simulink model "is95fwdchendtoend"  (Simulink 4.00)
settings: Solver=VariableStepDiscrete  SolverMode=SingleTasking  StartTime=0.0  StopTime=600  RelTol=1e-3  AbsTol=1e-6
undefined symbols (not defined in the file): Fs, magnitude
libraries: cdmalib x14, dspsrcs2 x13, dspbuff2 x5, dspxfrm2 x3, dspstat2 x3, dspsnks2 x3, dspmtrx2 x2, commsink x2, commchan x2
settings Model: RequirementInfo=9  Creator=pc  LastModifiedBy=akansal  SaveTime=off  SaveOutput=off  LimitDataPoints=off  ExtModeTrigMode=oneshot  ExtModeArmWhenConnect=off  BlockReductionOpt=off

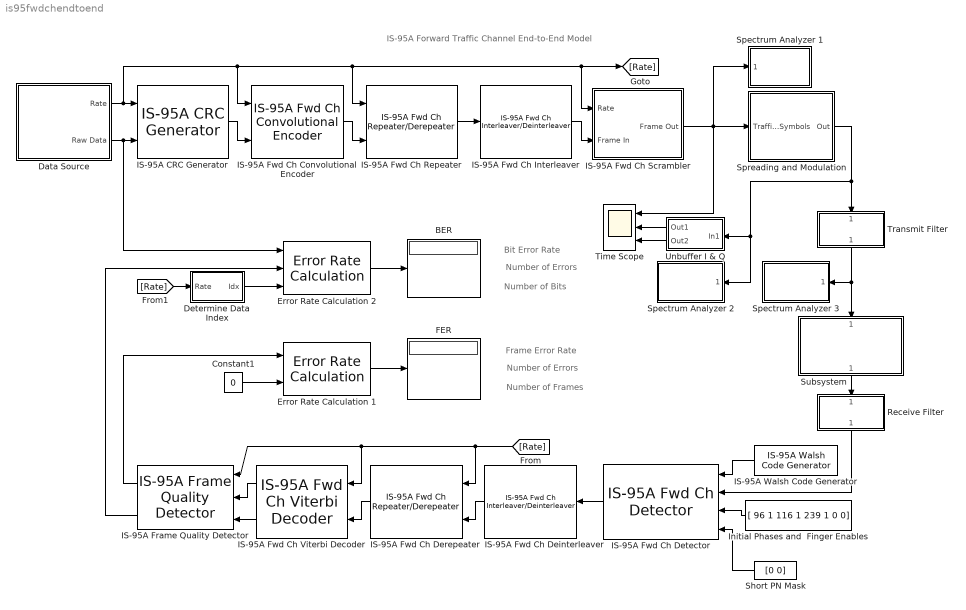
== system is95fwdchendtoend ==
  note: IS-95A Forward Traffic Channel
      | End-to-End Model
  note: Frame Error Rate
  note: Number of Errors
  note: Number of Frames
  note: Bit Error Rate
  note: Number of Errors
  note: Number of Bits
  BER : Display
      settings: Format=short
  Constant1 : Constant  Value=0
  Data Source : Subsystem
      settings: RTWFcnNameOpts=Auto  RTWFileNameOpts=Auto
  Determine Data Index : Subsystem  mask(Determine Data Index){rateSet=Rate Set I}
      mask prompts: rateSet "Rate set:"
      mask help: Deterime index of valid data in the frame based upon rate set and rate input.
      mask init:
      | if(rateSet==1)
      | % --- Rate Set 1
      |    R1F = buffer(1:172,268);
      |    R1H = buffer(1:80,268);
      |    R1Q = buffer(1:40,268);
      |    R1E = buffer(1:16,268);
      |    idxMat = [R1F R1H R1Q R1E];
      | else
      |    % --- Rate Set 2
      |    R2F = [1:268]';
      |    R2H = buffer(1:126,268);
      |    R2Q = buffer(1:56,268);
      |    R2E = buffer(1:22,268);
      |    idxMat = [R2F R2H R2Q R2E];
      | end;
      settings: RTWFcnNameOpts=Auto  RTWFileNameOpts=Auto
      mask StyleString: popup(Rate Set I|Rate Set II)
  Error Rate Calculation 1 : commsink/Error Rate Calculation  N=0  st_delay=4  cp_mode=Entire frame  subframe=[]  PMode=Port  WsName=ErrorVec  RsMode2=off
  Error Rate Calculation 2 : commsink/Error Rate Calculation  N=2*268  st_delay=2*268  cp_mode=Select samples from port  subframe=[]  PMode=Port  WsName=ErrorVec  RsMode2=off
  FER : Display
      settings: Format=short
  IS-95A CRC Generator : cdmalib/IS-95A Common/IS-95A CRC Generator  rate_set=Rate Set I  ch_type=Traffic
  IS-95A Frame Quality Detector : cdmalib/IS-95A Common/IS-95A Frame Quality  Detector  Orientation=left  rateSet=Rate Set I  chType=Traffic  rate2_metric=0.9*1.5  rate3_metric=0.85*1.5
  IS-95A Fwd Ch Convolutional Encoder : cdmalib/IS-95A Base Station Transmitter/IS-95A Fwd Ch Convolutional Encoder  rate_set=Rate Set I  ch_type=Traffic  enc_state=[]
  IS-95A Fwd Ch Deinterleaver : cdmalib/IS-95A Base Station Transmitter/IS-95A Fwd Ch Interleaver//Deinterleaver  Orientation=left  ch_type=Traffic  int_select=Deinterleaver
  IS-95A Fwd Ch Derepeater : cdmalib/IS-95A Base Station Transmitter/IS-95A Fwd Ch Repeater//Derepeater  Orientation=left  rate_set=Rate Set I  ch_type=Traffic  rep_select=Derepeater
  IS-95A Fwd Ch Interleaver : cdmalib/IS-95A Base Station Transmitter/IS-95A Fwd Ch Interleaver//Deinterleaver  ch_type=Traffic  int_select=Interleaver
  IS-95A Fwd Ch Repeater : cdmalib/IS-95A Base Station Transmitter/IS-95A Fwd Ch Repeater//Derepeater  rate_set=Rate Set I  ch_type=Traffic  rep_select=Repeater
  IS-95A Fwd Ch Scrambler : Subsystem  mask(IS-95A Fwd Ch Scrambler){rate_set=Rate Set I, chType=Traffic}
      mask prompts: rate_set "Rate Set"; chType "Channel Type"
      mask help: Performs scrambling of the Forward Traffic channel data by the long code and the insertion of power bits in the data.
      settings: RTWFcnNameOpts=Auto  RTWFileNameOpts=Auto
      mask Help: web(cdmaweb);
      mask StyleString: popup(Rate Set I|Rate Set II),popup(Sync|Paging|Traffic)
  IS-95A Fwd Ch Viterbi Decoder : cdmalib/IS-95A Mobile Station Receiver/IS-95A Fwd Ch Viterbi Decoder  Orientation=left  rateSet=Rate Set I  chType=Traffic  traceBackLenRatio=1  decodeLenRatio=1
  IS-95A Fwd Ch Detector : cdmalib/IS-95A Mobile Station Receiver/IS-95A Fwd Ch Detector  Orientation=left  rateSet=Rate Set I  numSymb=1  wlshOrd=6  rake_buff_size=3  rake_oversamp=8  sampTime=1/(50*384)
  IS-95A Walsh Code Generator : cdmalib/IS-95A Common/IS-95A Walsh Code Generator  Orientation=left  wlshOrd=6  wlshIndices=38  st=1/50/384
  Initial Phases and  Finger Enables : Constant  Orientation=left  Value=[ 96 1 116 1 239 1 0 0]
  Receive Filter : Subsystem  Orientation=down  mask{N=1}
      mask prompts: N "Interpolation factor:"
      mask init:
      | load txfiltx8.mat;
      | h = (TxFiltCoefx8*N)/8;
      settings: RTWFcnNameOpts=Auto  RTWFileNameOpts=Auto
      mask Display: plot( 1:prod( size( h)), h);
  Short PN Mask : Constant  Orientation=left  Value=[0 0]
  Spectrum Analyzer 1 : Subsystem
      settings: RTWFcnNameOpts=Auto  RTWFileNameOpts=Auto
      mask Display: disp('Spectrum\nAnalyzer');
  Spectrum Analyzer 2 : Subsystem  Orientation=left
      settings: RTWFcnNameOpts=Auto  RTWFileNameOpts=Auto
      mask Display: disp('Spectrum\nAnalyzer');
  Spectrum Analyzer 3 : Subsystem  Orientation=left
      settings: RTWFcnNameOpts=Auto  RTWFileNameOpts=Auto
      mask Display: disp('Spectrum\nAnalyzer');
  Spreading and Modulation : Subsystem
      settings: RTWFcnNameOpts=Auto  RTWFileNameOpts=Auto
      mask Display: disp('Combine with\nSync & Paging\n---\nSS Modulate')
  Subsystem : Subsystem  Orientation=down
      settings: RTWFcnNameOpts=Auto  RTWFileNameOpts=Auto
      mask Display: disp('Rayleigh Multipath\n and  AWGN\nChannel')
  Time Scope : Scope  NumInputPorts=3
      settings: TimeRange=0.001041666666666667  YMin=-3~-3~-3  YMax=3~3~3  SaveToWorkspace=off  SaveName=ScopeData  DataFormat=Structure  LimitDataPoints=on  MaxDataPoints=5000
  Transmit Filter : Subsystem  Orientation=down  mask{N=8}
      mask prompts: N "Interpolation factor:"
      mask init:
      | load txfiltx8.mat;
      | h = (TxFiltCoefx8*N)/8;
      settings: RTWFcnNameOpts=Auto  RTWFileNameOpts=Auto
      mask Display: plot( 1:prod( size( h)), h);
  Unbuffer I & Q : Subsystem  Orientation=left
      settings: RTWFcnNameOpts=Auto  RTWFileNameOpts=Auto
      mask Display: disp('Unbuffer\nI & Q');
  wires:
  Error Rate Calculation 2/1 -> BER/1
  [Rate] -> Determine Data Index/1(Rate)
  Error Rate Calculation 1/1 -> FER/1
  Constant1/1 -> Error Rate Calculation 1/2
  Determine Data Index/1(Idx) -> Error Rate Calculation 2/3
  Subsystem/1("  ") -> Receive Filter/1("   ")
  Initial Phases and  Finger Enables/1 -> IS-95A Fwd Ch Detector/3
  IS-95A Walsh Code Generator/1 -> IS-95A Fwd Ch Detector/1
  Short PN Mask/1 -> IS-95A Fwd Ch Detector/4
  IS-95A Fwd Ch Deinterleaver/1 -> IS-95A Fwd Ch Derepeater/2
  IS-95A Fwd Ch Derepeater/1 -> IS-95A Fwd Ch Viterbi Decoder/2
  IS-95A Fwd Ch Viterbi Decoder/1 -> IS-95A Frame Quality Detector/2
  IS-95A Fwd Ch Viterbi Decoder/2 -> IS-95A Frame Quality Detector/3
  IS-95A Fwd Ch Detector/1 -> IS-95A Fwd Ch Deinterleaver/1
  Receive Filter/1(" ") -> IS-95A Fwd Ch Detector/2
  IS-95A Frame Quality Detector/1 -> Error Rate Calculation 1/1
  IS-95A Frame Quality Detector/2 -> Error Rate Calculation 2/2
  [Rate] -> IS-95A Fwd Ch Derepeater/1, IS-95A Frame Quality Detector/1, IS-95A Fwd Ch Viterbi Decoder/1
  IS-95A Fwd Ch Repeater/1 -> IS-95A Fwd Ch Interleaver/1
  IS-95A Fwd Ch Convolutional Encoder/1 -> IS-95A Fwd Ch Repeater/2
  Data Source/1(Rate) -> IS-95A Fwd Ch Convolutional Encoder/1, IS-95A Fwd Ch Repeater/1, [Rate], IS-95A Fwd Ch Scrambler/1(Rate), IS-95A CRC Generator/1
  IS-95A Fwd Ch Interleaver/1 -> IS-95A Fwd Ch Scrambler/2(Frame In)
  IS-95A CRC Generator/1 -> IS-95A Fwd Ch Convolutional Encoder/2
  Data Source/2(Raw Data) -> IS-95A CRC Generator/2, Error Rate Calculation 2/1
  IS-95A Fwd Ch Scrambler/1(" Frame Out") -> Spreading and Modulation/1(Traffic Symbols), Spectrum Analyzer 1/1(" "), Time Scope/1
  Spreading and Modulation/1("Out ") -> Transmit Filter/1("   "), Spectrum Analyzer 2/1(" "), Unbuffer I & Q/1(In1)
  Transmit Filter/1(" ") -> Subsystem/1(" "), Spectrum Analyzer 3/1(" ")
  Unbuffer I & Q/1(Out1) -> Time Scope/2
  Unbuffer I & Q/2(Out2) -> Time Scope/3

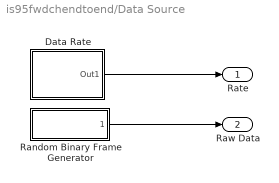
== system is95fwdchendtoend/Data Source ==
  Data Rate : Subsystem  mask{rate=Full}
      mask prompts: rate "Data Rate"
      settings: RTWFcnNameOpts=Auto  RTWFileNameOpts=Auto
      mask StyleString: popup(Full|Half|Quarter|One-Eighth)
      mask Display: disp('Base Station \nTransmitter\nData Rate')
  Random Binary Frame Generator : Subsystem  mask(Random binary frame generator){seed=1234, Ts=1/(50*268), N=268}
      mask prompts: seed "Initial seed:"; Ts "Sample time (sec):"; N "Output frame size:"
      mask help:
      | Generate a random frame of binary integers. The output frame period is
      | (Sample time) * (Output frame size).
      settings: RTWFcnNameOpts=Auto  RTWFileNameOpts=Auto
      mask Display: plot(0,0,100,100,[95,90,90,80,80,60,60,30,30,20,20,10,10,5],[25,25,75,75,25,25,75,75,25,25,75,75,25,25]);
  Rate : Outport  Port=1  InitialOutput=0
  Raw Data : Outport  Port=2  InitialOutput=0
  wires:
  Data Rate/1(Out1) -> Rate/1
  Random Binary Frame Generator/1(" ") -> Raw Data/1

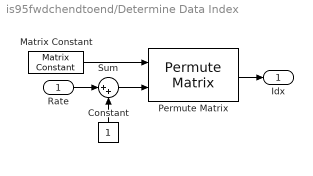
== system is95fwdchendtoend/Determine Data Index ==
  Rate : Inport  Port=1
  Constant : Constant  Orientation=up  Value=1
  Matrix Constant : dspmtrx2/Matrix Constant  M=idxMat
  Permute Matrix : dspmtrx2/Permute Matrix  mode=Columns  errmode=Clip Index  cols=4
  Sum : Sum  Inputs=|++  SaturateOnIntegerOverflow=on
  Idx : Outport  Port=1
  wires:
  Constant/1 -> Sum/2
  Matrix Constant/1 -> Permute Matrix/1
  Permute Matrix/1 -> Idx/1
  Sum/1 -> Permute Matrix/2
  Rate/1 -> Sum/1

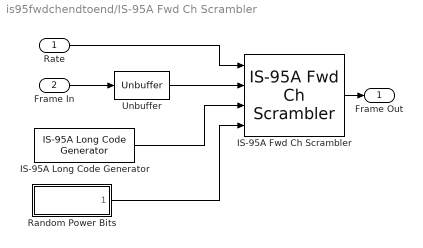
== system is95fwdchendtoend/IS-95A Fwd Ch Scrambler ==
  Rate : Inport  Port=1
  Frame In : Inport  Port=2
  IS-95A Fwd Ch Scrambler : cdmalib/IS-95A Base Station Transmitter/IS-95A Fwd Ch Scrambler  rate_set=Rate Set I  chType=Traffic
  IS-95A Long Code Generator : cdmalib/IS-95A Common/IS-95A Long Code Generator  num_symb=1  tx_lc_dec_ratio=64  tx_lc_init_mask=2^41  tx_lc_init_state=2^41  tx_sample_time=1/(50*384)
  Random Power Bits : Subsystem  mask(Random binary frame generator){seed=956742, Ts=1/50/16, N=1}
      mask prompts: seed "Initial seed:"; Ts "Sample time (sec):"; N "Ouput frame size:"
      settings: RTWFcnNameOpts=Auto  RTWFileNameOpts=Auto
      mask Display: plot(0,0,100,100,[95,90,90,80,80,60,60,30,30,20,20,10,10,5],[25,25,75,75,25,25,75,75,25,25,75,75,25,25]);
  Unbuffer : dspbuff2/Unbuffer  ic=0  num_chans=1
  " Frame Out" : Outport  Port=1  InitialOutput=0
  wires:
  Rate/1 -> IS-95A Fwd Ch Scrambler/1
  IS-95A Fwd Ch Scrambler/1 -> " Frame Out"/1
  Random Power Bits/1(" ") -> IS-95A Fwd Ch Scrambler/4
  Frame In/1 -> Unbuffer/1
  Unbuffer/1 -> IS-95A Fwd Ch Scrambler/2
  IS-95A Long Code Generator/1 -> IS-95A Fwd Ch Scrambler/3

== system is95fwdchendtoend/Receive Filter ==
  "   " : Inport  Port=1
  FIR Interpolation : Subsystem  mask(FIR Interpolation){h=h, L=N, frame=on, numChans=1, framing=Maintain input frame rate}
      mask prompts: h "FIR filter coefficients:"; L "Interpolation factor:"; frame "Frame-based inputs"; numChans "Number of channels:"
      mask help: Upsample input signal by an integer factor, then apply an FIR filter. Implemented using an efficient polyphase interpolation structure. The filter coefficients are scaled by the interpolation factor.
      mask init:
      | outputBufInitCond = 0;
      | [str,numChans] = dspblkupfir('setup1',numChans);
      | [h,framing,str]= dspblkupfir('setup2',h,L,framing);
      settings: RTWFcnNameOpts=Auto  RTWFileNameOpts=Auto
      mask Help: web(dspbhelp);
      mask StyleString: edit,edit,checkbox,edit,popup(Maintain input frame size|Maintain input frame rate)
      mask CallbackString: ||dspblkupfir||
      mask Display: disp(str)
  " " : Outport  Port=1
  wires:
  "   "/1 -> FIR Interpolation/1(in_1)
  FIR Interpolation/1(out_1) -> " "/1

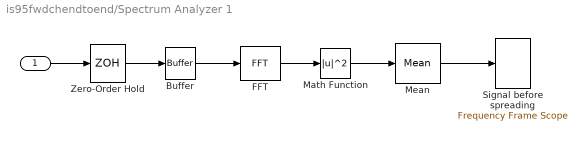
== system is95fwdchendtoend/Spectrum Analyzer 1 ==
  " " : Inport  Port=1
  Buffer : dspbuff2/Buffer  N=1024  V=0  ic=0
  FFT : dspxfrm2/FFT  nchans=1
  Math Function : Math  Operator=magnitude^2  OutputSignalType=auto
  Mean : dspstat2/Mean  run=on  reset=off  frame=off  nchans=1
  Signal before spreading : dspsnks2/Frequency Frame Scope  Domain=Frequency  XLabel=Samples  XUnits=Hertz  XRange=[-Fs/2...Fs/2]  XIncr=-1  YLabel=Magnitude, dB  YUnits=dB  HorizSpan=1  NChans=1  AxisParams=on  FigPos=[339 599 602 134]  AxisGrid=on  AxisZoom=on  FrameNumber=off  AxisLegend=off  Memory=off  LineParams=off
      settings: YMin=-10  YMax=100
  Zero-Order Hold : ZeroOrderHold  SampleTime=1/50/384/64
  wires:
  Zero-Order Hold/1 -> Buffer/1
  " "/1 -> Zero-Order Hold/1
  Buffer/1 -> FFT/1
  FFT/1 -> Math Function/1
  Math Function/1 -> Mean/1
  Mean/1 -> Signal before spreading/1

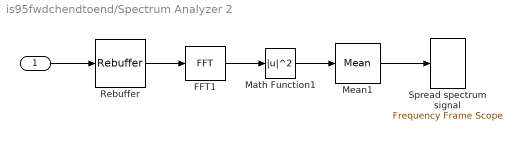
== system is95fwdchendtoend/Spectrum Analyzer 2 ==
  " " : Inport  Port=1
  FFT1 : dspxfrm2/FFT  nchans=1
  Math Function1 : Math  Operator=magnitude^2  OutputSignalType=auto
  Mean1 : dspstat2/Mean  run=on  reset=off  frame=off  nchans=1
  Rebuffer : dspbuff2/Rebuffer  Specify_Out_Size=on  N=1024  V=0  ic=0  frame=on  num_chans=1
  Spread spectrum signal : dspsnks2/Frequency Frame Scope  Domain=Frequency  XLabel=Samples  XUnits=Hertz  XRange=[-Fs/2...Fs/2]  XIncr=-1  YLabel=Magnitude, dB  YUnits=dB  HorizSpan=1  NChans=1  AxisParams=on  FigPos=[339 439 602 134]  AxisGrid=on  AxisZoom=on  FrameNumber=off  AxisLegend=off  Memory=off  LineParams=off
      settings: YMin=-10  YMax=100
  wires:
  " "/1 -> Rebuffer/1
  Rebuffer/1 -> FFT1/1
  Mean1/1 -> Spread spectrum signal/1
  FFT1/1 -> Math Function1/1
  Math Function1/1 -> Mean1/1

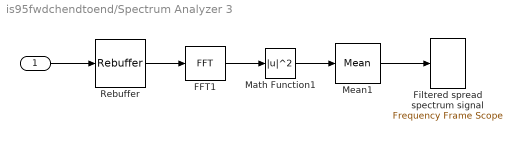
== system is95fwdchendtoend/Spectrum Analyzer 3 ==
  " " : Inport  Port=1
  FFT1 : dspxfrm2/FFT  nchans=1
  Filtered spread spectrum signal : dspsnks2/Frequency Frame Scope  Domain=Frequency  XLabel=Samples  XUnits=Hertz  XRange=[-Fs/2...Fs/2]  XIncr=-1  YLabel=Magnitude, dB  YUnits=dB  HorizSpan=1  NChans=1  AxisParams=on  FigPos=[339 281 602 134]  AxisGrid=on  AxisZoom=on  FrameNumber=off  AxisLegend=off  Memory=off  LineParams=off
      settings: YMin=-10  YMax=100
  Math Function1 : Math  Operator=magnitude^2  OutputSignalType=auto
  Mean1 : dspstat2/Mean  run=on  reset=off  frame=off  nchans=1
  Rebuffer : dspbuff2/Rebuffer  Specify_Out_Size=on  N=8192  V=0  ic=0  frame=on  num_chans=1
  wires:
  Math Function1/1 -> Mean1/1
  FFT1/1 -> Math Function1/1
  Mean1/1 -> Filtered spread spectrum signal/1
  Rebuffer/1 -> FFT1/1
  " "/1 -> Rebuffer/1

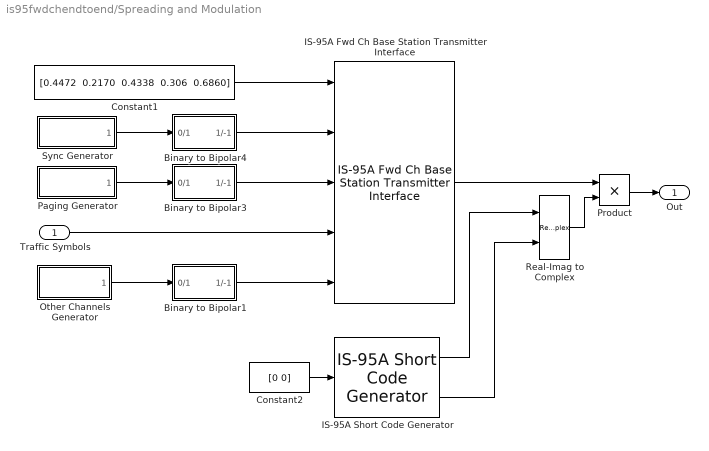
== system is95fwdchendtoend/Spreading and Modulation ==
  Traffic Symbols : Inport  Port=1
  Binary to Bipolar1 : Subsystem
      settings: RTWFcnNameOpts=Auto  RTWFileNameOpts=Auto
      mask Type: Binary to Bipolar Transformation
      mask Description: Binary to Bipolar Transformation.
  Binary to Bipolar3 : Subsystem
      settings: RTWFcnNameOpts=Auto  RTWFileNameOpts=Auto
      mask Type: Binary to Bipolar Transformation
      mask Description: Binary to Bipolar Transformation.
  Binary to Bipolar4 : Subsystem
      settings: RTWFcnNameOpts=Auto  RTWFileNameOpts=Auto
      mask Type: Binary to Bipolar Transformation
      mask Description: Binary to Bipolar Transformation.
  Constant1 : Constant  Value="[0.4472  0.2170  0.4338  0.306  0.6860]"
  Constant2 : Constant  Value=[0 0]
  IS-95A Fwd Ch Base Station Transmitter Interface : cdmalib/IS-95A Base Station Transmitter/IS-95A Fwd Ch Base Station Transmitter Interface  paging_rate=Full  wlshOrd=6  wlsh_indices=[0 32 47 38 23]  sampTime=1/(50*384)
  IS-95A Short Code Generator : cdmalib/IS-95A Common/IS-95A Short Code Generator  numOut=64  sampTime=1/(50*384)
  Other Channels Generator : Subsystem  mask(Random binary frame generator){seed=98767657, Ts=1/(50*384), N=1}
      mask prompts: seed "Initial seed:"; Ts "Sample time (sec):"; N "Output frame size:"
      mask help:
      | Generate a random frame of binary integers. The output frame period is
      | (Sample time) * (Output frame size).
      settings: RTWFcnNameOpts=Auto  RTWFileNameOpts=Auto
      mask Display: plot(0,0,100,100,[95,90,90,80,80,60,60,30,30,20,20,10,10,5],[25,25,75,75,25,25,75,75,25,25,75,75,25,25]);
  Paging Generator : Subsystem  mask(Random binary frame generator){seed=76767, Ts=1/(50*384), N=1}
      mask prompts: seed "Initial seed:"; Ts "Sample time (sec):"; N "Output frame size:"
      mask help:
      | Generate a random frame of binary integers. The output frame period is
      | (Sample time) * (Output frame size).
      settings: RTWFcnNameOpts=Auto  RTWFileNameOpts=Auto
      mask Display: plot(0,0,100,100,[95,90,90,80,80,60,60,30,30,20,20,10,10,5],[25,25,75,75,25,25,75,75,25,25,75,75,25,25]);
  Product : Product  Inputs=2  Multiplication=Element-wise(.*)  SaturateOnIntegerOverflow=on
  Real-Imag to Complex : RealImagToComplex  Input=RealAndImag  ConstantPart=0
  Sync Generator : Subsystem  mask(Random binary frame generator){seed=465789, Ts=4 * 1/(50*384), N=1}
      mask prompts: seed "Initial seed:"; Ts "Sample time (sec):"; N "Output frame size:"
      mask help:
      | Generate a random frame of binary integers. The output frame period is
      | (Sample time) * (Output frame size).
      settings: RTWFcnNameOpts=Auto  RTWFileNameOpts=Auto
      mask Display: plot(0,0,100,100,[95,90,90,80,80,60,60,30,30,20,20,10,10,5],[25,25,75,75,25,25,75,75,25,25,75,75,25,25]);
  "Out " : Outport  Port=1  InitialOutput=0
  wires:
  Sync Generator/1(" ") -> Binary to Bipolar4/1(0/1)
  Paging Generator/1(" ") -> Binary to Bipolar3/1(0/1)
  Other Channels Generator/1(" ") -> Binary to Bipolar1/1(0/1)
  Constant2/1 -> IS-95A Short Code Generator/1
  Constant1/1 -> IS-95A Fwd Ch Base Station Transmitter Interface/1
  Binary to Bipolar4/1(1/-1) -> IS-95A Fwd Ch Base Station Transmitter Interface/2
  Binary to Bipolar3/1(1/-1) -> IS-95A Fwd Ch Base Station Transmitter Interface/3
  Traffic Symbols/1 -> IS-95A Fwd Ch Base Station Transmitter Interface/4
  Binary to Bipolar1/1(1/-1) -> IS-95A Fwd Ch Base Station Transmitter Interface/5
  Real-Imag to Complex/1 -> Product/2
  IS-95A Fwd Ch Base Station Transmitter Interface/1 -> Product/1
  Product/1 -> "Out "/1
  IS-95A Short Code Generator/1 -> Real-Imag to Complex/1
  IS-95A Short Code Generator/2 -> Real-Imag to Complex/2

== system is95fwdchendtoend/Subsystem ==
  " " : Inport  Port=1
  AWGN Channel : commchan/AWGN channel  seed=17583  noiseMode="Signal to noise ratio  (Es/No)"  EsNodB=-3.0  SNRdB=4.3-9  Ps=2  Tsym=1/1228800  variance=1  FrameBased=on  nChans=1
  Multipath Rayleigh Fading : commchan/Multipath Rayleigh Fading  Fd=175.92  simTs=1/(1228800*8)  delayVec=[0 2e-6 14.5e-6]  gainVecdB=[0 0 -3]  normGain=on  Seed=1234
  "  " : Outport  Port=1
  wires:
  AWGN Channel/1 -> "  "/1
  " "/1 -> Multipath Rayleigh Fading/1
  Multipath Rayleigh Fading/1 -> AWGN Channel/1

== system is95fwdchendtoend/Transmit Filter ==
  "   " : Inport  Port=1
  FIR Interpolation : Subsystem  mask(FIR Interpolation){h=h, L=N, frame=on, numChans=1, framing=Maintain input frame rate}
      mask prompts: h "FIR filter coefficients:"; L "Interpolation factor:"; frame "Frame-based inputs"; numChans "Number of channels:"
      mask help: Upsample input signal by an integer factor, then apply an FIR filter. Implemented using an efficient polyphase interpolation structure. The filter coefficients are scaled by the interpolation factor.
      mask init:
      | outputBufInitCond = 0;
      | [str,numChans] = dspblkupfir('setup1',numChans);
      | [h,framing,str]= dspblkupfir('setup2',h,L,framing);
      settings: RTWFcnNameOpts=Auto  RTWFileNameOpts=Auto
      mask Help: web(dspbhelp);
      mask StyleString: edit,edit,checkbox,edit,popup(Maintain input frame size|Maintain input frame rate)
      mask CallbackString: ||dspblkupfir||
      mask Display: disp(str)
  " " : Outport  Port=1
  wires:
  FIR Interpolation/1(out_1) -> " "/1
  "   "/1 -> FIR Interpolation/1(in_1)

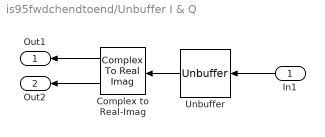
== system is95fwdchendtoend/Unbuffer I & Q ==
  In1 : Inport  Orientation=left  Port=1
  Complex to Real-Imag : ComplexToRealImag  Orientation=left  Output=RealAndImag
  Unbuffer : dspbuff2/Unbuffer  Orientation=left  ic=0  num_chans=1
  Out1 : Outport  Orientation=left  Port=1
  Out2 : Outport  Orientation=left  Port=2
  wires:
  Unbuffer/1 -> Complex to Real-Imag/1
  Complex to Real-Imag/1 -> Out1/1
  Complex to Real-Imag/2 -> Out2/1
  In1/1 -> Unbuffer/1

== system is95fwdchendtoend/Data Source/Data Rate ==
  Rate : Constant  Value=rate-1
  Zero-Order Hold3 : ZeroOrderHold  SampleTime=1/50
  Out1 : Outport  Port=1  InitialOutput=0
  wires:
  Zero-Order Hold3/1 -> Out1/1
  Rate/1 -> Zero-Order Hold3/1

== system is95fwdchendtoend/Data Source/Random Binary Frame Generator ==
  Discrete Constant : dspsrcs2/Discrete Constant  Value=0  Ts=Ts*N
  Random Source : dspsrcs2/Random Source  SrcType=Gaussian  Min=0  Max=1  Mean=0  Var=1  Seed=seed  Inherit=off  SampMode=Discrete  SampTime=Ts  SampFrame=N  OutComplex=Real
  Relational Operator : RelationalOperator  Operator=>
  " " : Outport  Port=1
  wires:
  Random Source/1 -> Relational Operator/1
  Discrete Constant/1 -> Relational Operator/2
  Relational Operator/1 -> " "/1

== system is95fwdchendtoend/IS-95A Fwd Ch Scrambler/Random Power Bits ==
  Discrete Constant : dspsrcs2/Discrete Constant  Value=0  Ts=Ts*N
  Random Source : dspsrcs2/Random Source  SrcType=Gaussian  Min=0  Max=1  Mean=0  Var=1  Seed=seed  Inherit=off  SampMode=Discrete  SampTime=Ts  SampFrame=N  OutComplex=Real
  Relational Operator : RelationalOperator  Operator=>
  " " : Outport  Port=1
  wires:
  Random Source/1 -> Relational Operator/1
  Discrete Constant/1 -> Relational Operator/2
  Relational Operator/1 -> " "/1

== system is95fwdchendtoend/Receive Filter/FIR Interpolation ==
  in_1 : Inport  Port=1
  upfir : S-Function  FunctionName=sdspupfir  Parameters=h,L,numChans,framing,outputBufInitCond  PortCounts=[]  SFunctionModules=''
  out_1 : Outport  Port=1  InitialOutput=0
  wires:
  upfir/1 -> out_1/1
  in_1/1 -> upfir/1

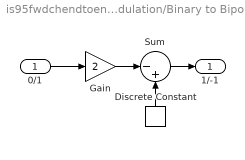
== system is95fwdchendtoend/Spreading and Modulation/Binary to Bipolar1 ==
  0/1 : Inport  Port=1
  Discrete Constant : dspsrcs2/Discrete Constant  Orientation=up  Value=1  Ts=1/(50*384)
  Gain : Gain  Gain=2  Multiplication=Element-wise(K.*u)  SaturateOnIntegerOverflow=on
  Sum : Sum  Inputs=|-+  SaturateOnIntegerOverflow=on
  1/-1 : Outport  Port=1  InitialOutput=0
  wires:
  Discrete Constant/1 -> Sum/2
  0/1/1 -> Gain/1
  Gain/1 -> Sum/1
  Sum/1 -> 1/-1/1

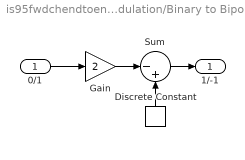
== system is95fwdchendtoend/Spreading and Modulation/Binary to Bipolar3 ==
  0/1 : Inport  Port=1
  Discrete Constant : dspsrcs2/Discrete Constant  Orientation=up  Value=1  Ts=1/(50*384)
  Gain : Gain  Gain=2  Multiplication=Element-wise(K.*u)  SaturateOnIntegerOverflow=on
  Sum : Sum  Inputs=|-+  SaturateOnIntegerOverflow=on
  1/-1 : Outport  Port=1  InitialOutput=0
  wires:
  Sum/1 -> 1/-1/1
  Gain/1 -> Sum/1
  0/1/1 -> Gain/1
  Discrete Constant/1 -> Sum/2

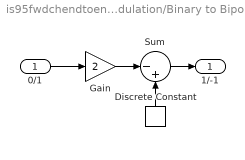
== system is95fwdchendtoend/Spreading and Modulation/Binary to Bipolar4 ==
  0/1 : Inport  Port=1
  Discrete Constant : dspsrcs2/Discrete Constant  Orientation=up  Value=1  Ts=4 * 1/(50*384)
  Gain : Gain  Gain=2  Multiplication=Element-wise(K.*u)  SaturateOnIntegerOverflow=on
  Sum : Sum  Inputs=|-+  SaturateOnIntegerOverflow=on
  1/-1 : Outport  Port=1  InitialOutput=0
  wires:
  Sum/1 -> 1/-1/1
  Gain/1 -> Sum/1
  0/1/1 -> Gain/1
  Discrete Constant/1 -> Sum/2

== system is95fwdchendtoend/Spreading and Modulation/Other Channels Generator ==
  Discrete Constant : dspsrcs2/Discrete Constant  Value=0  Ts=Ts*N
  Random Source : dspsrcs2/Random Source  SrcType=Gaussian  Min=0  Max=1  Mean=0  Var=1  Seed=seed  Inherit=off  SampMode=Discrete  SampTime=Ts  SampFrame=N  OutComplex=Real
  Relational Operator : RelationalOperator  Operator=>
  " " : Outport  Port=1
  wires:
  Random Source/1 -> Relational Operator/1
  Discrete Constant/1 -> Relational Operator/2
  Relational Operator/1 -> " "/1

== system is95fwdchendtoend/Spreading and Modulation/Paging Generator ==
  Discrete Constant : dspsrcs2/Discrete Constant  Value=0  Ts=Ts*N
  Random Source : dspsrcs2/Random Source  SrcType=Gaussian  Min=0  Max=1  Mean=0  Var=1  Seed=seed  Inherit=off  SampMode=Discrete  SampTime=Ts  SampFrame=N  OutComplex=Real
  Relational Operator : RelationalOperator  Operator=>
  " " : Outport  Port=1
  wires:
  Random Source/1 -> Relational Operator/1
  Discrete Constant/1 -> Relational Operator/2
  Relational Operator/1 -> " "/1

== system is95fwdchendtoend/Spreading and Modulation/Sync Generator ==
  Discrete Constant : dspsrcs2/Discrete Constant  Value=0  Ts=Ts*N
  Random Source : dspsrcs2/Random Source  SrcType=Gaussian  Min=0  Max=1  Mean=0  Var=1  Seed=seed  Inherit=off  SampMode=Discrete  SampTime=Ts  SampFrame=N  OutComplex=Real
  Relational Operator : RelationalOperator  Operator=>
  " " : Outport  Port=1
  wires:
  Relational Operator/1 -> " "/1
  Discrete Constant/1 -> Relational Operator/2
  Random Source/1 -> Relational Operator/1

== system is95fwdchendtoend/Transmit Filter/FIR Interpolation ==
  in_1 : Inport  Port=1
  upfir : S-Function  FunctionName=sdspupfir  Parameters=h,L,numChans,framing,outputBufInitCond  PortCounts=[]  SFunctionModules=''
  out_1 : Outport  Port=1  InitialOutput=0
  wires:
  in_1/1 -> upfir/1
  upfir/1 -> out_1/1
